simulink model "Prob_3_DM_II"  (R2025a)
settings: Solver=VariableStepAuto  StartTime=0.0  StopTime=10.0  RelTol=1e-3
settings Model: Creator=claudelieber  LastModifiedBy=yugpn

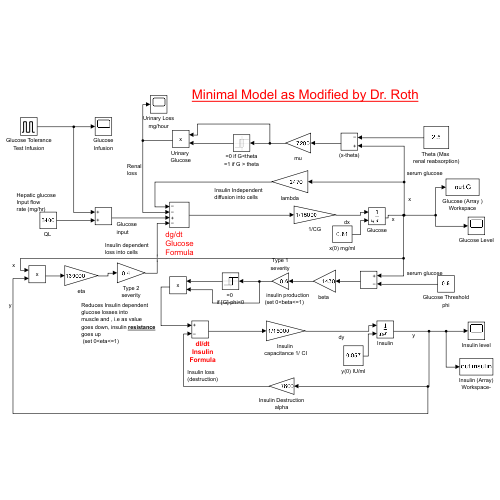
[thumbnail: Simulink's stored preview of the top-level diagram]
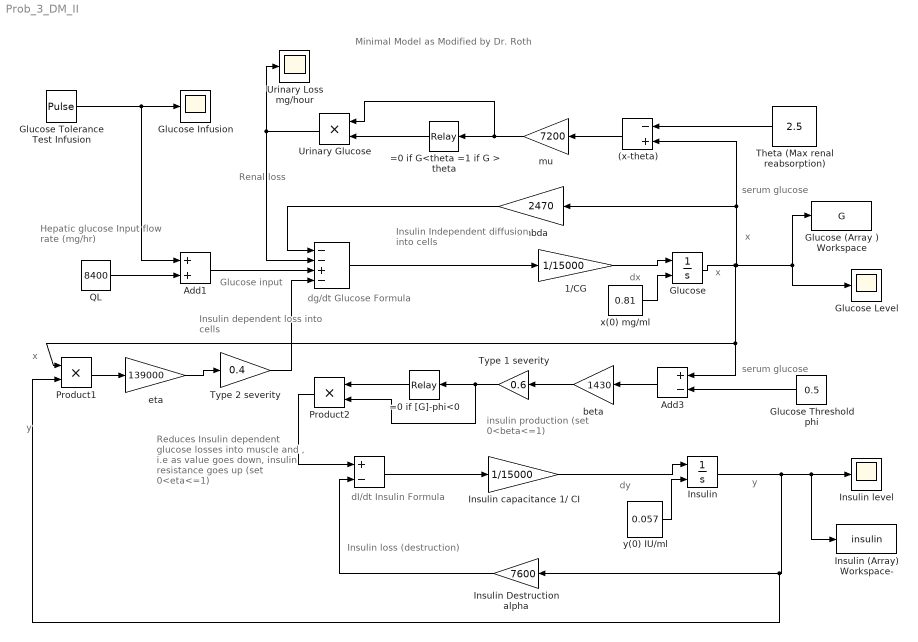
== system Prob_3_DM_II ==
  note: Renal
      | loss
  note: Minimal Model as Modified by Dr. Roth
  note: Glucose
      | input
  note: y
  note: Hepatic glucose
      | Input flow
      | rate (mg/hr)
  note: Insulin Independent
      | diffusion into cells
  note: dy
  note: insulin production
      | (set 0<beta<=1)
  note: Reduces Insulin dependent
      | glucose losses into
      | muscle and , i.e as value
      | goes down, insulin resistance
      | goes up
      | (set 0<eta<=1)
  note: dI/dt
      | Insulin
      | Formula
  note: x
  note: dg/dt
      | Glucose
      | Formula
  note: serum glucose
  note: serum glucose
  note: x
  note: y
  note: Insulin dependent
      | loss into cells
  note: x
  note: Insulin loss
      | (destruction)
  note: dx
  " " : Sum  Inputs=--+-
  " " : Sum  Inputs=+-
  (x-theta) : Sum  Inputs=-+
  1/CG : Gain  Gain=1/15000
  =0 if [G]-phi<0 : Relay  OnSwitchValue=0  OffSwitchValue=-0.0001
  =0 if G<theta =1 if G > theta : Relay  OnSwitchValue=0  OffSwitchValue=-0.00001
  Add1 : Sum
  Add3 : Sum  Inputs=+-
  Glucose : Integrator  InitialConditionSource=external  InitialCondition=0.81
  Glucose Infusion : Scope
      settings: ActiveDisplayYMinimum=-1.2276276151838468  ActiveDisplayYMaximum=1.127228918584317  DataLoggingSaveFormat=Array
  Glucose (Array ) Workspace : ToWorkspace  VariableName=G  SampleTime=-1
  Glucose Level : Scope
      settings: ActiveDisplayYMinimum=0.72701525558169011  ActiveDisplayYMaximum=1.3272172493412124  DataLoggingVariableName=ScopeData2
  Glucose Threshold phi : Constant  Value=0.5
  Glucose Tolerance Test Infusion : DiscretePulseGenerator  PulseType=Time based  Amplitude=0  Period=10  PulseWidth=5
  Insulin : Integrator  InitialConditionSource=external  InitialCondition=0.055
  Insulin capacitance 1/ CI : Gain  Gain=1/15000
  Insulin (Array) Workspace- : ToWorkspace  VariableName=insulin  SampleTime=-1
  Insulin Destruction alpha : Gain  Gain=7600
  Insulin level : Scope
      settings: ActiveDisplayYMinimum=0.049416665518873387  ActiveDisplayYMaximum=0.085668403414165054  DataLoggingVariableName=ScopeData3  DataLoggingSaveFormat=Array
  Product1 : Product
  Product2 : Product
  "QL " : Constant  Value=8400
  Theta (Max renal reabsorption) : Constant  Value=2.5
  Type 1 severity : Gain  Gain=0.6
  Type 2 severity : Gain  Gain=0.4
  Urinary Glucose : Product
  Urinary Loss mg/hour : Scope
      settings: ActiveDisplayYMinimum=-1.1983222052132938  ActiveDisplayYMaximum=1.1730210392718903
  "beta " : Gain  Gain=1430
  "eta " : Gain  Gain=139000
  lambda : Gain  Gain=2470
  mu : Gain  Gain=7200
  x(0) mg/ml : Constant  Value=0.81
  y(0) IU/ml : Constant  Value=0.057
  wires:
  1/CG/1 -> Glucose/1
  Theta (Max renal reabsorption)/1 -> (x-theta)/1
  x(0) mg/ml/1 -> Glucose/2
  =0 if [G]-phi<0/1 -> Product2/1
  Insulin/1 -> Product1/2, Insulin Destruction alpha/1, Insulin (Array) Workspace-/1, Insulin level/1
  Add3/1 -> "beta "/1
  Urinary Glucose/1 -> " "/2, Urinary Loss mg/hour/1
  Glucose Tolerance Test Infusion/1 -> Add1/1, Glucose Infusion/1
  Product1/1 -> "eta "/1
  "eta "/1 -> Type 2 severity/1
  " "/1 -> Insulin capacitance 1/ CI/1
  mu/1 -> Urinary Glucose/1, =0 if G<theta =1 if G > theta/1
  =0 if G<theta =1 if G > theta/1 -> Urinary Glucose/2
  Glucose/1 -> Product1/1, Add3/1, Glucose Level/1, Glucose (Array ) Workspace/1, (x-theta)/2, lambda/1
  Insulin capacitance 1/ CI/1 -> Insulin/1
  y(0) IU/ml/1 -> Insulin/2
  Glucose Threshold phi/1 -> Add3/2
  "QL "/1 -> Add1/2
  Type 2 severity/1 -> " "/4
  Add1/1 -> " "/3
  (x-theta)/1 -> mu/1
  Product2/1 -> " "/1
  lambda/1 -> " "/1
  " "/1 -> 1/CG/1
  "beta "/1 -> Type 1 severity/1
  Insulin Destruction alpha/1 -> " "/2
  Type 1 severity/1 -> Product2/2, =0 if [G]-phi<0/1
